simulink model "ReducingofBlockDiagram"  (R2018a)
settings: Solver=VariableStepAuto  StartTime=0.0  StopTime=10.0  RelTol=1e-3
undefined symbols (not defined in the file or in its folder): Controller, fm, Jm, km, km2, La, Ra, s2LaJm, sJm, sLa
settings Model: Creator=Neo  LastModifiedBy=Neo

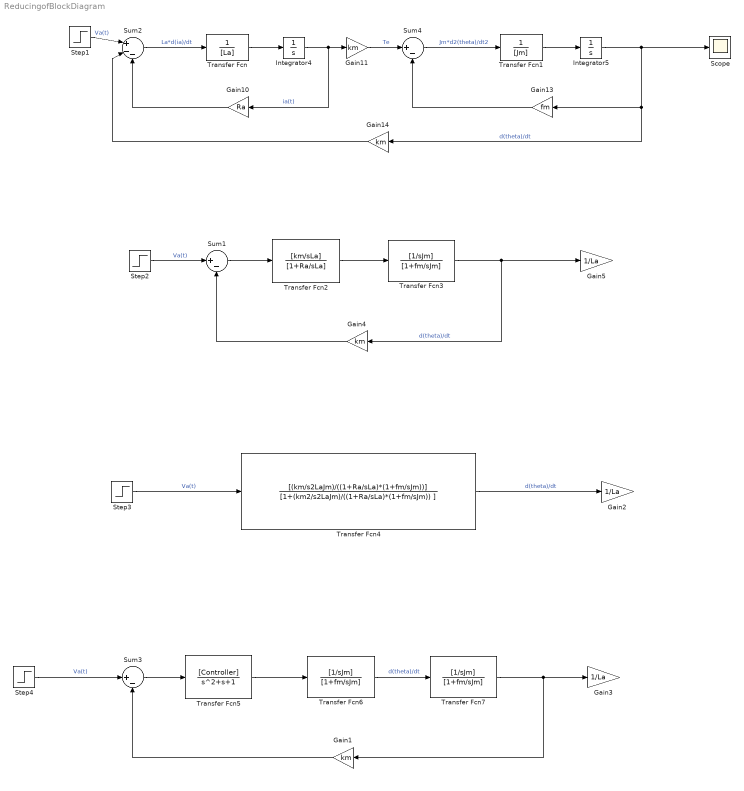
== system ReducingofBlockDiagram ==
  Gain{1,4,11,14} (4 alike) : Gain  Gain=km
  Gain10 : Gain  Gain=Ra
  Gain13 : Gain  Gain=fm
  Gain2 : Gain  Gain=1/La
  Gain3 : Gain  Gain=1/La
  Gain5 : Gain  Gain=1/La
  Integrator4 : Integrator
  Integrator5 : Integrator
  Scope : Scope
  Step{1..4} (4 alike) : Step  Time=0  After=10  SampleTime=0
  Sum1 : Sum  Inputs=|+-
  Sum2 : Sum  Inputs=|+--
  Sum3 : Sum  Inputs=|+-
  Sum4 : Sum  Inputs=|+-
  Transfer Fcn : TransferFcn  Denominator=[La]
  Transfer Fcn1 : TransferFcn  Denominator=[Jm]
  Transfer Fcn2 : TransferFcn  Numerator=[km/sLa]  Denominator=[1+Ra/sLa]
  Transfer Fcn3 : TransferFcn  Numerator=[1/sJm]  Denominator=[1+fm/sJm]
  Transfer Fcn4 : TransferFcn  Numerator=[(km/s2LaJm)/((1+Ra/sLa)*(1+fm/sJm))]  Denominator=[1+(km2/s2LaJm)/((1+Ra/sLa)*(1+fm/sJm)) ]
  Transfer Fcn5 : TransferFcn  Numerator=[Controller]  Denominator=[1 1 1]
  Transfer Fcn6 : TransferFcn  Numerator=[1/sJm]  Denominator=[1+fm/sJm]
  Transfer Fcn7 : TransferFcn  Numerator=[1/sJm]  Denominator=[1+fm/sJm]
  wires:
  Gain14/1 -> Sum2/2
  Step1/1 -> Sum2/1  "Va(t)"
  Gain13/1 -> Sum4/2
  Gain11/1 -> Sum4/1  "Te"
  Integrator5/1 -> Scope/1, Gain13/1, Gain14/1  "d(theta)/dt"
  Gain10/1 -> Sum2/3
  Integrator4/1 -> Gain11/1, Gain10/1  "ia(t)"
  Gain4/1 -> Sum1/2
  Step2/1 -> Sum1/1  "Va(t)"
  Sum2/1 -> Transfer Fcn/1  "La*d(ia)/dt"
  Transfer Fcn/1 -> Integrator4/1
  Sum4/1 -> Transfer Fcn1/1  "Jm*d2(theta)/dt2"
  Transfer Fcn1/1 -> Integrator5/1
  Sum1/1 -> Transfer Fcn2/1
  Transfer Fcn2/1 -> Transfer Fcn3/1
  Transfer Fcn3/1 -> Gain5/1, Gain4/1  "d(theta)/dt"
  Step3/1 -> Transfer Fcn4/1  "Va(t)"
  Transfer Fcn4/1 -> Gain2/1  "d(theta)/dt"
  Step4/1 -> Sum3/1  "Va(t)"
  Sum3/1 -> Transfer Fcn5/1
  Gain1/1 -> Sum3/2
  Transfer Fcn5/1 -> Transfer Fcn6/1
  Transfer Fcn6/1 -> Transfer Fcn7/1  "d(theta)/dt"
  Transfer Fcn7/1 -> Gain1/1, Gain3/1
